simulink model "advanced_modelError"  (R2023a)
settings: Solver=ode1  StartTime=0  StopTime=1200  FixedStep=0.002  RelTol=1e-3  EnableMultiTasking=on
values from neighbouring files (symbols this model uses):
  angleLim = pi/3    (= 1.0471975512)    [modelCompPlot.m]
  B = b*L*(K_v)^2 /J_xx    (= 0.042375883612)    [advanced_model_setup.m]    (also in brusselator.m = 2.15; cycle_detection.m = img2; cycle_detection_start.m = img2; demonstrateDetections.m = 2.15)
  cycleGain = 0.1    [advanced_model_setup.m]
  f_p = 1.3    [advanced_model_setup.m]    (also in modelCompPlot.m)
  f_r = 0.4    [advanced_model_setup.m]    (also in modelCompPlot.m)
  f_y = 0.175    [advanced_model_setup.m]    (also in modelCompPlot.m)
  g_p = 10.5    [advanced_model_setup.m]    (also in modelCompPlot.m)
  g_r = 5.2    [advanced_model_setup.m]    (also in modelCompPlot.m)
  I_xx = 0.0522    [advanced_model_setup.m]    (also in modelCompPlot.m; set_model_params.m; solveSyms3d_2.m = evalin('base', 'I_xx'))
  I_yy = 0.0522    [advanced_model_setup.m]    (also in modelCompPlot.m; set_model_params.m; solveSyms3d_2.m = evalin('base', 'I_yy'))
  I_zz = 0.1104    [advanced_model_setup.m]    (also in modelCompPlot.m; set_model_params.m; solveSyms3d_2.m = evalin('base', 'I_zz'))
  J = (J_yy - J_zz)/J_xx    (= -1)    [advanced_model_setup.m]    (also in modelCompPlot.m)
  J_r = J_inertia/J_xx    (= 0.00108695652174)    [advanced_model_setup.m]    (also in modelCompPlot.m; solveSyms3d.m = evalin('base', 'J_r'))
  Jp = 2*Jeq_prop    (= 0.0552224595625)    [modelCompPlot.m]    (also in set_model_params.m)
  Jr = 2*Jeq_prop    (= 0.0552224595625)    [modelCompPlot.m]    (also in set_model_params.m)
  k_T = 0.1188    [advanced_model_setup.m]    (also in modelCompPlot.m; set_model_params.m; solveSyms3d_2.m = evalin('base', 'k_T'))
  K_v = 54.945    [advanced_model_setup.m]    (also in modelCompPlot.m; solveSyms3d.m = evalin('base', 'K_v'))
  kd = 0.5    [advanced_model_setup.m]
  Kf = 0.1188    [modelCompPlot.m]    (also in set_model_params.m)
  kfr_p = 0.4*u2line/x5line    (= 0.285774113641)    [advanced_model_setup.m]    (also in modelCompPlot.m; set_model_params.m)
  kfr_r = 0.4*u1line/x4line    (= 0.285774113641)    [advanced_model_setup.m]    (also in modelCompPlot.m; set_model_params.m)
  L = 0.1969    [advanced_model_setup.m]    (also in modelCompPlot.m; set_model_params.m = 0.19685)
  l_a = 0.1968    [advanced_model_setup.m]    (also in modelCompPlot.m; set_model_params.m; solveSyms3d_2.m = evalin('base', 'l_a'))
  r = 0.2    [advanced_model_setup.m]    (also in gainScheduling.m = evalin('base', 'r'))
  sigma = 0    [modelCompPlot.m]
  skew = 1    [advanced_model_setup.m]
  V_bias = 12    [advanced_model_setup.m]    (also in modelCompPlot.m; set_model_params.m; solveSyms3d.m = evalin('base', 'V_bias'))
  velMax = 1000    [advanced_model_setup.m]
  VMAX_AMP = 24    [advanced_model_setup.m]    (also in modelCompPlot.m; set_model_params.m)
  wcf = 2 * pi * 20    (= 125.663706144)    [advanced_model_setup.m]    (also in modelCompPlot.m; set_model_params.m)
  Y = d*(K_v)^2 /J_zz    (= 0.0032609614876)    [advanced_model_setup.m]    (also in modelCompPlot.m; solveSyms3d.m = evalin('base', 'Y'))
  zetaf = 0.6    [advanced_model_setup.m]    (also in modelCompPlot.m; set_model_params.m)
libraries: simulink_extras x4, dspsrcs4 x1
settings Model: ExtModeTrigDuration=10000  Creator=kille  LastModifiedBy=Jacob
settings SolverCC: PositivePriorityOrder=on  AutoInsertRateTranBlk=on
settings DataIOCC: ReturnWorkspaceOutputs=off
settings OptimizationCC: LifeSpan=inf
settings DebuggingCC: UnconnectedInputMsg=warning  UnconnectedOutputMsg=warning  UnconnectedLineMsg=warning  ArithmeticOperatorsInVariantConditions=warning
settings ModelReferenceCC: EnableRefExpFcnMdlSchedulingChecks=on
settings SFSimCC: SimUseLocalCustomCode=off  CustomCodeUndefinedFunction=UseInterfaceOnly
settings RTWCC: Description=QUARC Win64 Target  SystemTargetFile=quarc_win64.tlc  TemplateMakefile=quarc_default_tmf  RTWUseLocalCustomCode=off
settings CodeAppCC: StateflowObjectComments=on
settings STFCustomTargetCC: TargetPreCompLibLocation=C:\PROGRA~3\QUARC\lib\2016a\win64\release  UseToolchainInfoCompliant=off  SystemTargetFile=quarc_win64.tlc
settings GRTTargetCC: TargetPreCompLibLocation=C:\PROGRA~3\QUARC\lib\2016a\win64\release  ParMdlRefBuildCompliant=off  CompOptLevelCompliant=off  CombineOutputUpdateFcns=off  MatFileLogging=off  CPPClassGenCompliant=off  GRTInterface=on  UseToolchainInfoCompliant=off  ExtMode=on  ExtModeMexFile=quarc_comm
settings ConfigComp: CovMetricSettings=dswe

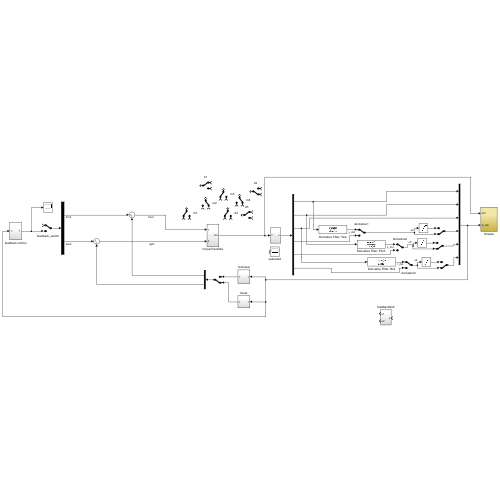
[thumbnail: Simulink's stored preview of the top-level diagram]
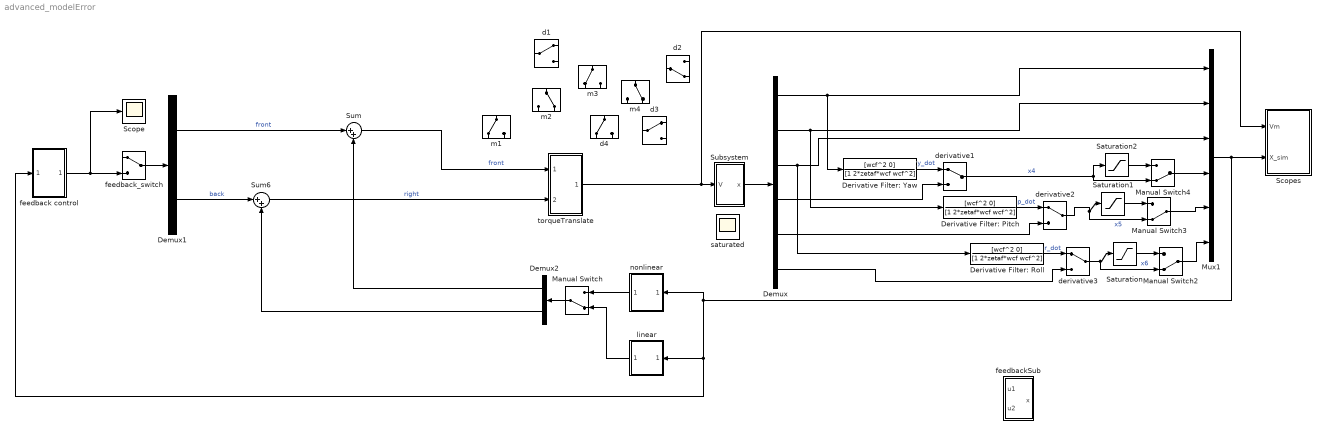
== system advanced_modelError ==
  Demux : Demux  Outputs=6
  Demux1 : Demux  Outputs=2
  Demux2 : Demux  Outputs=2
  Derivative Filter: Pitch : TransferFcn  Numerator=[wcf^2 0]  Denominator=[1 2*zetaf*wcf wcf^2]
  Derivative Filter: Roll : TransferFcn  Numerator=[wcf^2 0]  Denominator=[1 2*zetaf*wcf wcf^2]
  Derivative Filter: Yaw : TransferFcn  Numerator=[wcf^2 0]  Denominator=[1 2*zetaf*wcf wcf^2]
  Manual Switch{,2..4} (4 alike) : ManualSwitch  CurrentSetting=0
  Mux1 : Mux  Inputs=6
  Saturation : Saturate  UpperLimit=velMax  LowerLimit=-velMax
  Saturation1 : Saturate  UpperLimit=velMax  LowerLimit=-velMax
  Saturation2 : Saturate  UpperLimit=velMax  LowerLimit=-velMax
  Scope : Scope
  Scopes : Subsystem
  Subsystem : Subsystem
  Sum : Sum  Inputs=|++
  Sum6 : Sum  Inputs=|++
  d1 : ManualSwitch
  d2 : ManualSwitch  CurrentSetting=0
  d3 : ManualSwitch
  d4 : ManualSwitch
  derivative1 : ManualSwitch
  derivative2 : ManualSwitch
  derivative3 : ManualSwitch
  feedback control : Subsystem
  feedbackSub : Subsystem
  feedback_switch : ManualSwitch
  linear : Subsystem
  m1 : ManualSwitch
  m2 : ManualSwitch  CurrentSetting=0
  m3 : ManualSwitch
  m4 : ManualSwitch  CurrentSetting=0
  nonlinear : Subsystem
  saturated : Scope
  torqueTranslate : Subsystem
  wires:
  Sum6/1 -> torqueTranslate/2(Input)  "right"
  Sum/1 -> torqueTranslate/1(In1)  "front"
  derivative2/1 -> Manual Switch3/2, Saturation1/1  "x5"
  Derivative Filter: Pitch/1 -> derivative2/1  "p_dot"
  Saturation2/1 -> Manual Switch4/1
  Saturation1/1 -> Manual Switch3/1
  Saturation/1 -> Manual Switch2/1
  Demux/4 -> derivative1/2
  derivative1/1 -> Saturation2/1, Manual Switch4/2  "x4"
  derivative3/1 -> Manual Switch2/2, Saturation/1  "x6"
  Derivative Filter: Roll/1 -> derivative3/1  "r_dot"
  Derivative Filter: Yaw/1 -> derivative1/1  "y_dot"
  Subsystem/1(x) -> Demux/1
  Manual Switch4/1 -> Mux1/4
  Manual Switch3/1 -> Mux1/5
  Manual Switch2/1 -> Mux1/6
  Demux/1 -> Derivative Filter: Yaw/1, Mux1/1
  Demux/2 -> Derivative Filter: Pitch/1, Mux1/2
  Demux/3 -> Derivative Filter: Roll/1, Mux1/3
  Demux/5 -> derivative2/2
  Demux/6 -> derivative3/2
  Demux1/1 -> Sum/1  "front"
  Demux1/2 -> Sum6/1  "back"
  feedback_switch/1 -> Demux1/1
  feedback control/1(Out1) -> Scope/1, feedback_switch/2
  Demux2/1 -> Sum/2
  Demux2/2 -> Sum6/2
  Manual Switch/1 -> Demux2/1
  nonlinear/1(Out1) -> Manual Switch/1
  linear/1(Out1) -> Manual Switch/2
  Mux1/1 -> Scopes/2(X_sim), linear/1(Input), feedback control/1(In1), nonlinear/1(Input)
  torqueTranslate/1(Vm) -> Scopes/1(Vm), Subsystem/1(V)

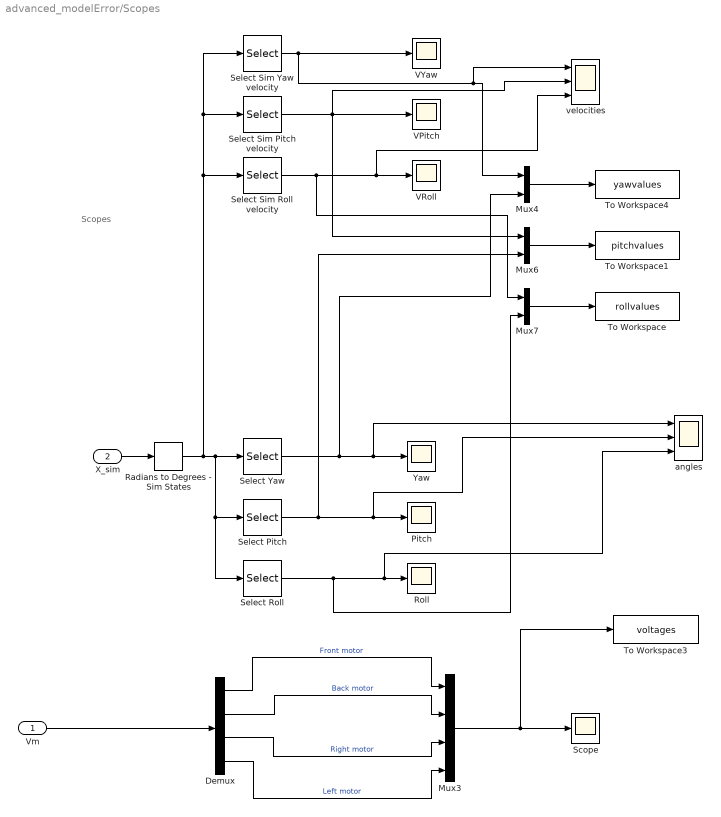
== system advanced_modelError/Scopes ==
  note: Scopes
  Vm : Inport
  X_sim : Inport  Port=2
  Demux : Demux
  Mux3 : Mux
  Mux4 : Mux  Inputs=2
  Mux6 : Mux  Inputs=2
  Mux7 : Mux  Inputs=2
  Pitch : Scope
  Radians to Degrees - Sim States : simulink_extras/Transformations/Radians to Degrees
  Roll : Scope
  Scope : Scope
  Select Pitch : Selector  InputPortWidth=6  IndexOptions=Index vector (dialog)  Indices=2  OutputSizes=1
  Select Roll : Selector  InputPortWidth=6  IndexOptions=Index vector (dialog)  Indices=3  OutputSizes=1
  Select Sim Pitch velocity : Selector  InputPortWidth=6  IndexOptions=Index vector (dialog)  Indices=5  OutputSizes=1
  Select Sim Roll velocity : Selector  InputPortWidth=6  IndexOptions=Index vector (dialog)  Indices=6  OutputSizes=1
  Select Sim Yaw velocity : Selector  InputPortWidth=6  IndexOptions=Index vector (dialog)  Indices=4  OutputSizes=1
  Select Yaw : Selector  InputPortWidth=6  IndexOptions=Index vector (dialog)  Indices=1  OutputSizes=1
  To Workspace : ToWorkspace  VariableName=rollvalues  SampleTime=-1
  To Workspace1 : ToWorkspace  VariableName=pitchvalues  SampleTime=-1
  To Workspace3 : ToWorkspace  VariableName=voltages  SampleTime=-1
  To Workspace4 : ToWorkspace  VariableName=yawvalues  SampleTime=-1
  VPitch : Scope
  VRoll : Scope
  VYaw : Scope
  Yaw : Scope
  angles : Scope  NumInputPorts=3
  velocities : Scope  NumInputPorts=3
  wires:
  Select Roll/1 -> angles/3, Roll/1, Mux7/2
  Radians to Degrees - Sim States/1 -> Select Sim Roll velocity/1, Select Sim Pitch velocity/1, Select Sim Yaw velocity/1, Select Roll/1, Select Pitch/1, Select Yaw/1
  Select Pitch/1 -> angles/2, Pitch/1, Mux6/2
  X_sim/1 -> Radians to Degrees - Sim States/1
  Demux/1 -> Mux3/1  "Front motor"
  Demux/2 -> Mux3/2  "Back motor"
  Demux/3 -> Mux3/3  "Right motor"
  Demux/4 -> Mux3/4  "Left motor"
  Vm/1 -> Demux/1
  Select Sim Yaw velocity/1 -> VYaw/1, velocities/1, Mux4/1
  Select Sim Roll velocity/1 -> velocities/3, VRoll/1, Mux7/1
  Select Sim Pitch velocity/1 -> Mux6/1, velocities/2, VPitch/1
  Mux4/1 -> To Workspace4/1
  Mux6/1 -> To Workspace1/1
  Mux7/1 -> To Workspace/1
  Mux3/1 -> To Workspace3/1, Scope/1
  Select Yaw/1 -> angles/1, Yaw/1, Mux4/2

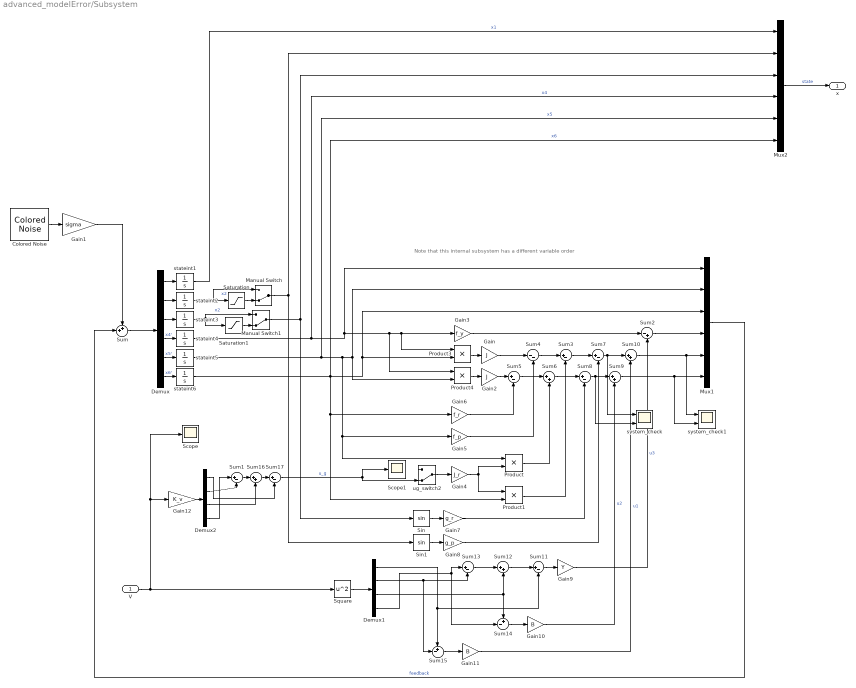
== system advanced_modelError/Subsystem ==
  note: Note that this internal subsystem has a different variable order
  V : Inport
  Colored Noise : dspsrcs4/Colored Noise  Color=white  InverseFrequencyPower=1  BoundedOutput=off  NumChannels=6  OutputDataType=double  SamplesPerFrame=1  SampleTime=1  RandomStream=mt19937ar with seed  Seed=67  SimulateUsing=Interpreted execution
  Demux : Demux  Outputs=6
  Demux1 : Demux
  Demux2 : Demux
  Gain : Gain  Gain=J
  Gain1 : Gain  Gain=sigma
  Gain10 : Gain  Gain=B
  Gain11 : Gain  Gain=B
  Gain12 : Gain  Gain=K_v
  Gain2 : Gain  Gain=J
  Gain3 : Gain  Gain=f_y
  Gain4 : Gain  Gain=J_r
  Gain5 : Gain  Gain=f_p
  Gain6 : Gain  Gain=f_r
  Gain7 : Gain  Gain=g_r
  Gain8 : Gain  Gain=g_p
  Gain9 : Gain  Gain=Y
  Manual Switch : ManualSwitch  CurrentSetting=0
  Manual Switch1 : ManualSwitch  CurrentSetting=0
  Mux1 : Mux  Inputs=6
  Mux2 : Mux  Inputs=6
  Product{,1,3..4} (4 alike) : Product
  Saturation : Saturate  UpperLimit=angleLim  LowerLimit=-angleLim
  Saturation1 : Saturate  UpperLimit=angleLim  LowerLimit=-angleLim
  Scope : Scope
  Scope1 : Scope
  Sin : Trigonometry
  Sin1 : Trigonometry
  Square : Math  Operator=square
  Sum : Sum  Inputs=++|
  Sum{1,3,5,7..8,11,13,17} (8 alike) : Sum  Inputs=|+-
  Sum{6,9..10,12,16} (5 alike) : Sum  Inputs=|++
  Sum14 : Sum  Inputs=+-|
  Sum15 : Sum  Inputs=+-|
  Sum2 : Sum  Inputs=|-+
  Sum4 : Sum  Inputs=|--
  stateint1 : Integrator  InitialCondition=0.034907
  stateint2 : Integrator  InitialCondition=0.034907
  stateint3 : Integrator  InitialCondition=0.034907
  stateint4 : Integrator
  stateint5 : Integrator
  stateint6 : Integrator
  system_check : Scope  NumInputPorts=2
  system_check1 : Scope  NumInputPorts=2
  ug_switch2 : ManualSwitch  CurrentSetting=0
  x : Outport
  wires:
  stateint5/1 -> Mux2/5, Gain5/1, Product/1, Mux1/2, Product4/2  "x5"
  stateint4/1 -> Mux2/4, Mux1/1, Product4/1, Product3/1, Gain3/1  "x4"
  Demux/1 -> stateint1/1
  stateint6/1 -> Mux2/6, Gain6/1, Product1/2, Mux1/3, Product3/2  "x6"
  Demux/6 -> stateint6/1  "x6'"
  Demux/5 -> stateint5/1  "x5'"
  Demux/2 -> stateint2/1
  Demux/3 -> stateint3/1
  Demux/4 -> stateint4/1  "x4'"
  Product3/1 -> Gain/1
  Product4/1 -> Gain2/1
  Colored Noise/1 -> Gain1/1
  Sum/1 -> Demux/1
  Gain1/1 -> Sum/1
  Gain3/1 -> Sum2/1
  Gain4/1 -> Product1/1, Product/2
  Sum17/1 -> ug_switch2/2, Scope1/1  "u_g"
  Gain/1 -> Sum4/1
  Gain2/1 -> Sum5/1
  Gain6/1 -> Sum5/2
  Gain5/1 -> Sum4/2
  Sum5/1 -> Sum6/1
  Product/1 -> Sum6/2
  Sum4/1 -> Sum3/1
  Sum6/1 -> Sum8/1
  Sum3/1 -> Sum7/1
  Gain7/1 -> Sum8/2
  Gain8/1 -> Sum7/2
  Sin/1 -> Gain7/1
  Sin1/1 -> Gain8/1
  Sum8/1 -> system_check/2, Sum9/1
  Sum7/1 -> system_check/1, Sum10/1
  Sum11/1 -> Gain9/1
  Gain9/1 -> Sum2/2  "u3"
  Square/1 -> Demux1/1
  Sum12/1 -> Sum11/1
  Sum13/1 -> Sum12/1
  Demux1/4 -> Sum13/1, Sum14/2
  Demux1/2 -> Sum13/2, Sum15/2
  Demux1/3 -> Sum12/2, Sum14/1
  Demux1/1 -> Sum15/1, Sum11/2
  Sum14/1 -> Gain10/1
  Sum15/1 -> Gain11/1
  Gain10/1 -> Sum9/2  "u2"
  Gain11/1 -> Sum10/2  "u1"
  Mux1/1 -> Sum/2  "feedback"
  V/1 -> Square/1, Scope/1, Gain12/1
  Gain12/1 -> Demux2/1
  Sum1/1 -> Sum16/1
  Sum16/1 -> Sum17/1
  Demux2/2 -> Sum1/2
  Demux2/3 -> Sum16/2
  Sum10/1 -> system_check1/1, Mux1/5
  Sum2/1 -> Mux1/4
  stateint2/1 -> Manual Switch/1, Saturation/1  "x2"
  Product1/1 -> Sum3/2
  Demux2/4 -> Sum1/1
  Demux2/1 -> Sum17/2
  stateint1/1 -> Mux2/1  "x1"
  Mux2/1 -> x/1  "state"
  Sum9/1 -> system_check1/2, Mux1/6
  ug_switch2/1 -> Gain4/1
  Manual Switch/1 -> Sin1/1, Mux2/2
  Saturation/1 -> Manual Switch/2
  Manual Switch1/1 -> Mux2/3, Sin/1
  stateint3/1 -> Saturation1/1, Manual Switch1/1  "x2"
  Saturation1/1 -> Manual Switch1/2

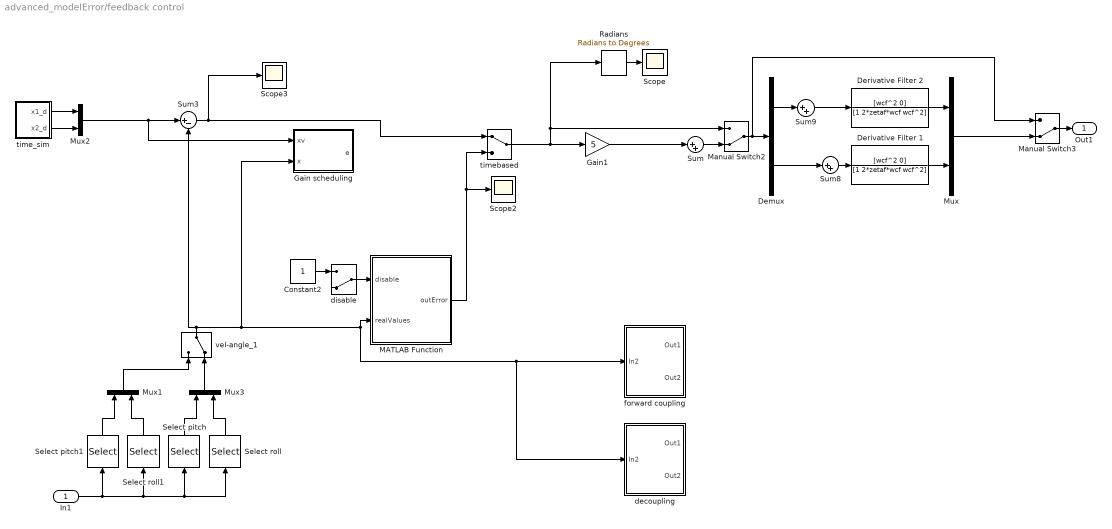
== system advanced_modelError/feedback control ==
  In1 : Inport
  Constant2 : Constant
  Demux : Demux  Outputs=2
  Derivative Filter 1 : TransferFcn  Numerator=[wcf^2 0]  Denominator=[1 2*zetaf*wcf wcf^2]
  Derivative Filter 2 : TransferFcn  Numerator=[wcf^2 0]  Denominator=[1 2*zetaf*wcf wcf^2]
  Gain scheduling : MATLAB Function  TreatAsAtomicUnit=on
  Gain1 : Gain  Gain=5
  MATLAB Function : MATLAB Function  TreatAsAtomicUnit=on
  Manual Switch2 : ManualSwitch  CurrentSetting=0
  Manual Switch3 : ManualSwitch  CurrentSetting=0
  Mux{,1..3} (4 alike) : Mux  Inputs=2
  Radians : simulink_extras/Transformations/Radians to Degrees
  Scope : Scope
  Scope2 : Scope
  Scope3 : Scope
  Select pitch : Selector  InputPortWidth=6  IndexOptions=Index vector (dialog)  Indices=2  OutputSizes=1
  Select pitch1 : Selector  InputPortWidth=6  IndexOptions=Index vector (dialog)  Indices=5  OutputSizes=1
  Select roll : Selector  InputPortWidth=6  IndexOptions=Index vector (dialog)  Indices=3  OutputSizes=1
  Select roll1 : Selector  InputPortWidth=6  IndexOptions=Index vector (dialog)  Indices=6  OutputSizes=1
  Sum : Sum  Inputs=|++
  Sum3 : Sum  Inputs=|+-
  Sum8 : Sum  Inputs=|++
  Sum9 : Sum  Inputs=|++
  decoupling : Subsystem
  disable : ManualSwitch  CurrentSetting=0
  forward coupling : Subsystem
  time_sim : Subsystem
  timebased : ManualSwitch
  vel-angle_1 : ManualSwitch  CurrentSetting=0
  Out1 : Outport
  wires:
  In1/1 -> Select roll/1, Select pitch/1, Select roll1/1, Select pitch1/1
  Select pitch/1 -> Mux3/1
  time_sim/1(x1_d) -> Mux2/1
  time_sim/2(x2_d) -> Mux2/2
  Select roll/1 -> Mux3/2
  MATLAB Function/1(outError) -> Scope2/1, timebased/2
  Sum/1 -> Manual Switch2/2
  Radians/1 -> Scope/1
  disable/1 -> MATLAB Function/1(disable)
  Constant2/1 -> disable/1
  Select roll1/1 -> Mux1/2
  Select pitch1/1 -> Mux1/1
  Mux1/1 -> vel-angle_1/1
  Mux3/1 -> vel-angle_1/2
  Mux2/1 -> Gain scheduling/1(xv), Sum3/1
  Derivative Filter 2/1 -> Mux/1
  Derivative Filter 1/1 -> Mux/2
  Manual Switch2/1 -> Manual Switch3/1, Demux/1
  Manual Switch3/1 -> Out1/1
  Demux/2 -> Sum8/1
  Mux/1 -> Manual Switch3/2
  vel-angle_1/1 -> Sum3/2, Gain scheduling/2(x), MATLAB Function/2(realValues), decoupling/1(In2), forward coupling/1(In2)
  Sum8/1 -> Derivative Filter 1/1
  Sum9/1 -> Derivative Filter 2/1
  Demux/1 -> Sum9/1
  Sum3/1 -> Scope3/1, timebased/1
  Gain1/1 -> Sum/1
  timebased/1 -> Manual Switch2/1, Radians/1, Gain1/1

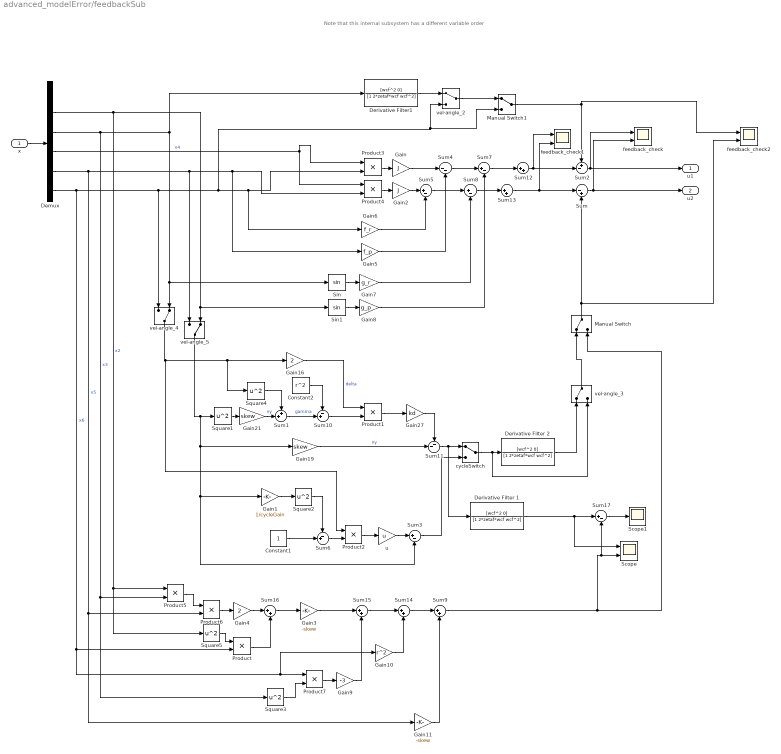
== system advanced_modelError/feedbackSub ==
  note: Note that this internal subsystem has a different variable order
  x : Inport
  Constant1 : Constant
  Constant2 : Constant  Value=r^2
  Demux : Demux  Outputs=6
  Derivative Filter 1 : TransferFcn  Numerator=[wcf^2 0]  Denominator=[1 2*zetaf*wcf wcf^2]
  Derivative Filter 2 : TransferFcn  Numerator=[wcf^2 0]  Denominator=[1 2*zetaf*wcf wcf^2]
  Derivative Filter1 : TransferFcn  Numerator=[wcf^2 0]  Denominator=[1 2*zetaf*wcf wcf^2]
  Gain : Gain  Gain=J
  Gain1 : Gain  Gain=1/cycleGain
  Gain10 : Gain  Gain=r^2
  Gain11 : Gain  Gain=-skew
  Gain16 : Gain  Gain=2
  Gain19 : Gain  Gain=skew
  Gain2 : Gain  Gain=J
  Gain21 : Gain  Gain=skew
  Gain27 : Gain  Gain=kd
  Gain3 : Gain  Gain=-skew
  Gain4 : Gain  Gain=2
  Gain5 : Gain  Gain=f_p
  Gain6 : Gain  Gain=f_r
  Gain7 : Gain  Gain=g_r
  Gain8 : Gain  Gain=g_p
  Gain9 : Gain  Gain=-3
  Manual Switch : ManualSwitch
  Manual Switch1 : ManualSwitch
  Product{,1..7} (8 alike) : Product
  Scope : Scope  NumInputPorts=2
  Scope1 : Scope
  Sin : Trigonometry
  Sin1 : Trigonometry
  Square{1..5} (5 alike) : Math  Operator=square
  Sum : Sum  Inputs=|-+
  Sum1 : Sum  Inputs=++|
  Sum10 : Sum  Inputs=-+|
  Sum11 : Sum  Inputs=--|
  Sum{9,12..16} (6 alike) : Sum  Inputs=|++
  Sum{3,5,7..8,17} (5 alike) : Sum  Inputs=|+-
  Sum2 : Sum  Inputs=+-|
  Sum4 : Sum  Inputs=|--
  Sum6 : Sum  Inputs=-+|
  cycleSwitch : ManualSwitch
  feedback_check : Scope  NumInputPorts=2
  feedback_check1 : Scope  NumInputPorts=2
  feedback_check2 : Scope  NumInputPorts=2
  u : Gain  Gain=u
  vel-angle_2 : ManualSwitch
  vel-angle_3 : ManualSwitch
  vel-angle_4 : ManualSwitch  CurrentSetting=0
  vel-angle_5 : ManualSwitch  CurrentSetting=0
  u1 : Outport
  u2 : Outport  Port=2
  wires:
  Demux/4 -> Product3/1, Product4/1  "x4"
  Product3/1 -> Gain/1
  Product4/1 -> Gain2/1
  Gain/1 -> Sum4/1
  Gain2/1 -> Sum5/1
  Gain6/1 -> Sum5/2
  Gain5/1 -> Sum4/2
  Sum4/1 -> Sum7/1
  Gain7/1 -> Sum8/2
  Gain8/1 -> Sum7/2
  Sin/1 -> Gain7/1
  Sin1/1 -> Gain8/1
  Demux/3 -> Square3/1, Product5/2, Derivative Filter1/1, Sin/1, vel-angle_4/2  "x3"
  Sum5/1 -> Sum8/1
  Derivative Filter 2/1 -> vel-angle_3/1
  Square1/1 -> Gain21/1
  Product1/1 -> Gain27/1
  Sum1/1 -> Sum10/2  "gamma"
  Constant2/1 -> Sum10/1
  Sum10/1 -> Product1/2
  Gain16/1 -> Product1/1  "delta"
  Gain21/1 -> Sum1/2  "ny"
  Square4/1 -> Sum1/1
  Gain27/1 -> Sum11/1
  Gain19/1 -> Sum11/2  "ny"
  Derivative Filter1/1 -> vel-angle_2/1
  Sum2/1 -> u1/1, feedback_check/1
  Sum/1 -> u2/1, feedback_check/2
  Sum6/1 -> Product2/2
  Demux/2 -> Sin1/1, vel-angle_5/2, Product5/1, Square5/1  "x2"
  Gain1/1 -> Square2/1
  u/1 -> Sum3/1
  Product2/1 -> u/1
  Square2/1 -> Sum6/1
  Constant1/1 -> Sum6/2
  Sum11/1 -> Derivative Filter 1/1, cycleSwitch/1
  cycleSwitch/1 -> vel-angle_3/2, Derivative Filter 2/1
  Sum3/1 -> cycleSwitch/2
  Demux/5 -> Gain11/1, Product6/2, Product4/2, Gain5/1, vel-angle_5/1  "x5"
  Demux/6 -> Gain10/1, Product7/1, Product/2, vel-angle_4/1, Manual Switch1/2, vel-angle_2/2, Gain6/1, Product3/2  "x6"
  Sum7/1 -> Sum12/1
  Sum8/1 -> Sum13/1
  Sum12/1 -> feedback_check1/1, Sum2/2
  Sum13/1 -> feedback_check1/2, Sum/1
  x/1 -> Demux/1
  vel-angle_4/1 -> Product2/1, Square4/1, Gain16/1
  vel-angle_5/1 -> Gain19/1, Gain1/1, Sum3/2, Square1/1
  Sum15/1 -> Sum14/1
  Sum14/1 -> Sum9/1
  Gain3/1 -> Sum15/1
  Sum16/1 -> Gain3/1
  Gain4/1 -> Sum16/1
  Product/1 -> Sum16/2
  Product6/1 -> Gain4/1
  Product5/1 -> Product6/1
  Product7/1 -> Gain9/1
  Gain9/1 -> Sum15/2
  Square3/1 -> Product7/2
  Gain10/1 -> Sum14/2
  Gain11/1 -> Sum9/2
  Square5/1 -> Product/1
  Sum17/1 -> Scope1/1
  Sum9/1 -> Scope/2, Sum17/2, Manual Switch/2
  Derivative Filter 1/1 -> Scope/1, Sum17/1
  Manual Switch/1 -> Sum/2, feedback_check2/2
  vel-angle_3/1 -> Manual Switch/1
  Manual Switch1/1 -> feedback_check2/1, Sum2/1
  vel-angle_2/1 -> Manual Switch1/1

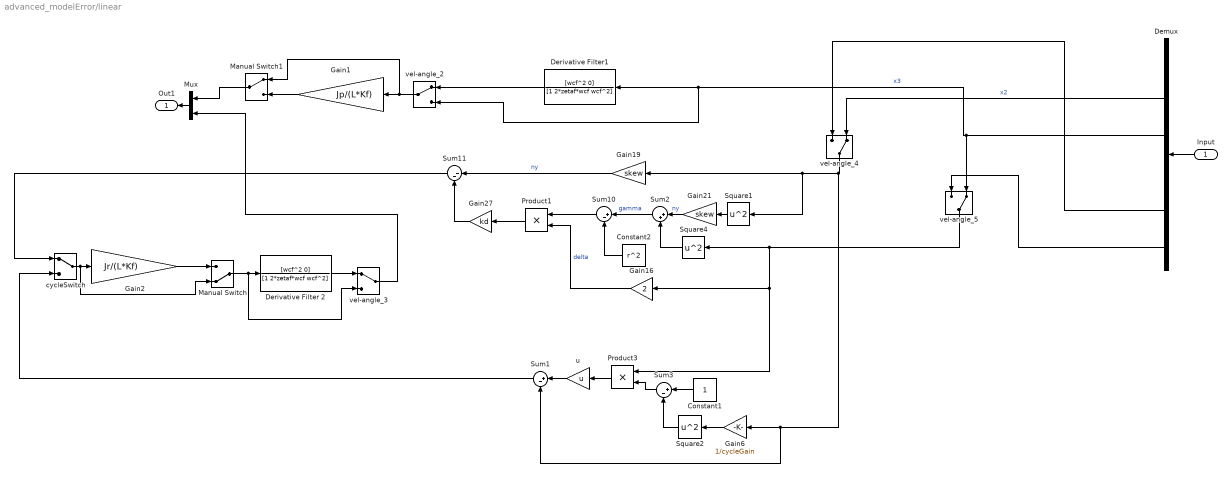
== system advanced_modelError/linear ==
  Input : Inport
  Constant1 : Constant
  Constant2 : Constant  Value=r^2
  Demux : Demux  Outputs=6
  Derivative Filter 2 : TransferFcn  Numerator=[wcf^2 0]  Denominator=[1 2*zetaf*wcf wcf^2]
  Derivative Filter1 : TransferFcn  Numerator=[wcf^2 0]  Denominator=[1 2*zetaf*wcf wcf^2]
  Gain1 : Gain  Gain=Jp/(L*Kf)
  Gain16 : Gain  Gain=2
  Gain19 : Gain  Gain=skew
  Gain2 : Gain  Gain=Jr/(L*Kf)
  Gain21 : Gain  Gain=skew
  Gain27 : Gain  Gain=kd
  Gain6 : Gain  Gain=1/cycleGain
  Manual Switch : ManualSwitch  CurrentSetting=0
  Manual Switch1 : ManualSwitch
  Mux : Mux  Inputs=2
  Product1 : Product
  Product3 : Product
  Square1 : Math  Operator=square
  Square2 : Math  Operator=square
  Square4 : Math  Operator=square
  Sum1 : Sum  Inputs=|+-
  Sum10 : Sum  Inputs=|+-
  Sum11 : Sum  Inputs=|--
  Sum2 : Sum  Inputs=|++
  Sum3 : Sum  Inputs=|+-
  cycleSwitch : ManualSwitch
  u : Gain  Gain=u
  vel-angle_2 : ManualSwitch
  vel-angle_3 : ManualSwitch
  vel-angle_4 : ManualSwitch  CurrentSetting=0
  vel-angle_5 : ManualSwitch  CurrentSetting=0
  Out1 : Outport
  wires:
  Square1/1 -> Gain21/1
  Product1/1 -> Gain27/1
  Square4/1 -> Sum2/2
  Gain19/1 -> Sum11/1  "ny"
  Sum2/1 -> Sum10/1  "gamma"
  Gain16/1 -> Product1/2  "delta"
  Sum10/1 -> Product1/1
  Gain27/1 -> Sum11/2
  Gain21/1 -> Sum2/1  "ny"
  Constant2/1 -> Sum10/2
  Sum1/1 -> cycleSwitch/2
  Demux/3 -> vel-angle_2/2, Derivative Filter1/1, vel-angle_5/2  "x3"
  u/1 -> Sum1/1
  Gain6/1 -> Square2/1
  Product3/1 -> u/1
  Constant1/1 -> Sum3/1
  Sum3/1 -> Product3/2
  Square2/1 -> Sum3/2
  Demux/2 -> vel-angle_4/2  "x2"
  Sum11/1 -> cycleSwitch/1
  Derivative Filter1/1 -> vel-angle_2/1
  vel-angle_2/1 -> Manual Switch1/1, Gain1/1
  cycleSwitch/1 -> Manual Switch/2, Gain2/1
  Derivative Filter 2/1 -> vel-angle_3/1
  Input/1 -> Demux/1
  vel-angle_4/1 -> Gain6/1, Sum1/2, Square1/1, Gain19/1
  Demux/5 -> vel-angle_4/1
  vel-angle_5/1 -> Product3/1, Gain16/1, Square4/1
  Demux/6 -> vel-angle_5/1
  Gain2/1 -> Manual Switch/1
  Manual Switch/1 -> vel-angle_3/2, Derivative Filter 2/1
  Gain1/1 -> Manual Switch1/2
  Manual Switch1/1 -> Mux/1
  vel-angle_3/1 -> Mux/2
  Mux/1 -> Out1/1

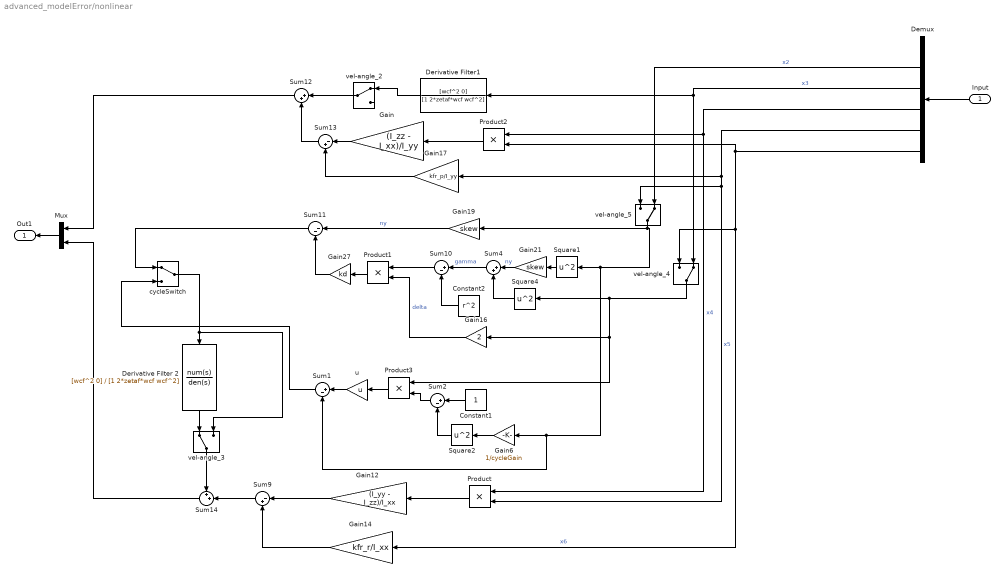
== system advanced_modelError/nonlinear ==
  Input : Inport
  Constant1 : Constant
  Constant2 : Constant  Value=r^2
  Demux : Demux  Outputs=6
  Derivative Filter 2 : TransferFcn  Numerator=[wcf^2 0]  Denominator=[1 2*zetaf*wcf wcf^2]
  Derivative Filter1 : TransferFcn  Numerator=[wcf^2 0]  Denominator=[1 2*zetaf*wcf wcf^2]
  Gain : Gain  Gain=(I_zz - I_xx)/I_yy
  Gain12 : Gain  Gain=(I_yy - I_zz)/I_xx
  Gain14 : Gain  Gain=kfr_r/I_xx
  Gain16 : Gain  Gain=2
  Gain17 : Gain  Gain=kfr_p/I_yy
  Gain19 : Gain  Gain=skew
  Gain21 : Gain  Gain=skew
  Gain27 : Gain  Gain=kd
  Gain6 : Gain  Gain=1/cycleGain
  Mux : Mux  Inputs=2
  Product{,1..3} (4 alike) : Product
  Square1 : Math  Operator=square
  Square2 : Math  Operator=square
  Square4 : Math  Operator=square
  Sum1 : Sum  Inputs=|+-
  Sum10 : Sum  Inputs=|+-
  Sum11 : Sum  Inputs=|--
  Sum12 : Sum  Inputs=|++
  Sum13 : Sum  Inputs=|-+
  Sum14 : Sum  Inputs=++|
  Sum2 : Sum  Inputs=|+-
  Sum4 : Sum  Inputs=|++
  Sum9 : Sum  Inputs=|-+
  cycleSwitch : ManualSwitch
  u : Gain  Gain=u
  vel-angle_2 : ManualSwitch
  vel-angle_3 : ManualSwitch
  vel-angle_4 : ManualSwitch  CurrentSetting=0
  vel-angle_5 : ManualSwitch  CurrentSetting=0
  Out1 : Outport
  wires:
  Derivative Filter1/1 -> vel-angle_2/1
  Gain17/1 -> Sum13/2
  Sum13/1 -> Sum12/2
  Demux/4 -> Product/1, Product2/1  "x4"
  Gain21/1 -> Sum4/1  "ny"
  Product2/1 -> Gain/1
  Demux/5 -> vel-angle_5/1, Product/2, Gain17/1  "x5"
  Gain27/1 -> Sum11/2
  Product/1 -> Gain12/1
  Constant2/1 -> Sum10/2
  Sum10/1 -> Product1/1
  Demux/6 -> vel-angle_4/1, Gain14/1, Product2/2  "x6"
  vel-angle_3/1 -> Sum14/1
  vel-angle_2/1 -> Sum12/1
  Sum4/1 -> Sum10/1  "gamma"
  Sum9/1 -> Sum14/2
  Square4/1 -> Sum4/2
  Gain12/1 -> Sum9/1
  Square1/1 -> Gain21/1
  Product1/1 -> Gain27/1
  Gain/1 -> Sum13/1
  Gain14/1 -> Sum9/2
  Sum12/1 -> Mux/1
  Gain19/1 -> Sum11/1  "ny"
  Gain16/1 -> Product1/2  "delta"
  Sum14/1 -> Mux/2
  Input/1 -> Demux/1
  Square2/1 -> Sum2/2
  Demux/2 -> vel-angle_5/2  "x2"
  Constant1/1 -> Sum2/1
  Sum2/1 -> Product3/2
  Product3/1 -> u/1
  Gain6/1 -> Square2/1
  Demux/3 -> Derivative Filter1/1, vel-angle_4/2  "x3"
  u/1 -> Sum1/1
  Sum11/1 -> cycleSwitch/1
  cycleSwitch/1 -> vel-angle_3/2, Derivative Filter 2/1
  Sum1/1 -> cycleSwitch/2
  vel-angle_4/1 -> Square4/1, Product3/1, Gain16/1
  vel-angle_5/1 -> Gain6/1, Sum1/2, Square1/1, Gain19/1
  Derivative Filter 2/1 -> vel-angle_3/1
  Mux/1 -> Out1/1

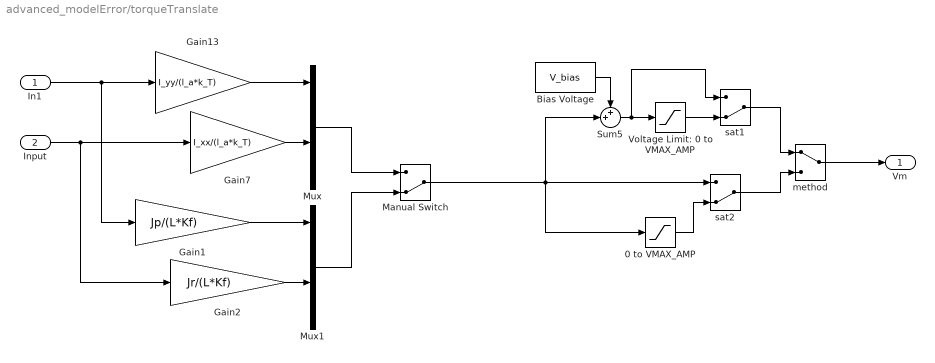
== system advanced_modelError/torqueTranslate ==
  In1 : Inport
  Input : Inport  Port=2
  0 to VMAX_AMP : Saturate  UpperLimit=VMAX_AMP  LowerLimit=0
  Bias Voltage : Constant  Value=V_bias
  Gain1 : Gain  Gain=Jp/(L*Kf)
  Gain13 : Gain  Gain=I_yy/(l_a*k_T)
  Gain2 : Gain  Gain=Jr/(L*Kf)
  Gain7 : Gain  Gain=I_xx/(l_a*k_T)
  Manual Switch : ManualSwitch  CurrentSetting=0
  Mux : Mux
  Mux1 : Mux
  Sum5 : Sum  Inputs=++|
  Voltage Limit: 0 to VMAX_AMP : Saturate  UpperLimit=VMAX_AMP  LowerLimit=0
  method : ManualSwitch  Tag=swt
  sat1 : ManualSwitch  CurrentSetting=0
  sat2 : ManualSwitch  CurrentSetting=0
  Vm : Outport
  wires:
  0 to VMAX_AMP/1 -> sat2/2
  Sum5/1 -> sat1/1, Voltage Limit: 0 to VMAX_AMP/1
  sat1/1 -> method/1
  Bias Voltage/1 -> Sum5/1
  Voltage Limit: 0 to VMAX_AMP/1 -> sat1/2
  sat2/1 -> method/2
  method/1 -> Vm/1
  Gain13/1 -> Mux/1
  In1/1 -> Gain13/1, Gain1/1
  Gain7/1 -> Mux/3
  Input/1 -> Gain7/1, Gain2/1
  Manual Switch/1 -> 0 to VMAX_AMP/1, Sum5/2, sat2/1
  Mux/1 -> Manual Switch/1
  Mux1/1 -> Manual Switch/2
  Gain1/1 -> Mux1/1
  Gain2/1 -> Mux1/3

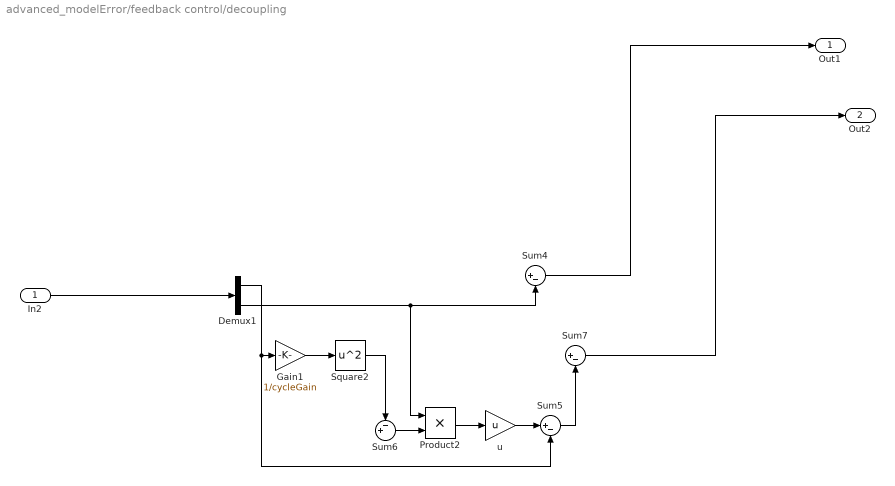
== system advanced_modelError/feedback control/decoupling ==
  In2 : Inport
  Demux1 : Demux  Outputs=2
  Gain1 : Gain  Gain=1/cycleGain
  Product2 : Product
  Square2 : Math  Operator=square
  Sum4 : Sum  Inputs=|+-
  Sum5 : Sum  Inputs=|+-
  Sum6 : Sum  Inputs=-+|
  Sum7 : Sum  Inputs=|+-
  u : Gain  Gain=u
  Out1 : Outport
  Out2 : Outport  Port=2
  wires:
  Sum5/1 -> Sum7/2
  Sum7/1 -> Out2/1
  Square2/1 -> Sum6/1
  u/1 -> Sum5/1
  Demux1/1 -> Sum5/2, Gain1/1
  Product2/1 -> u/1
  Demux1/2 -> Product2/1, Sum4/2
  Sum6/1 -> Product2/2
  Gain1/1 -> Square2/1
  In2/1 -> Demux1/1
  Sum4/1 -> Out1/1

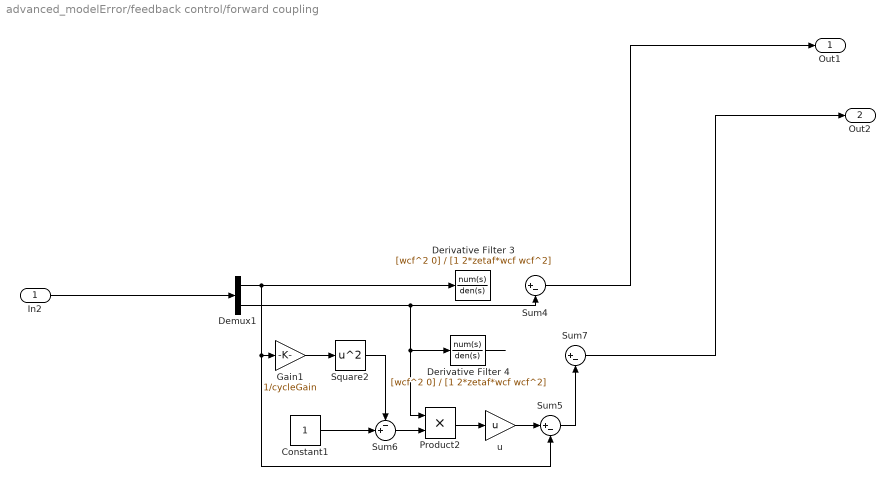
== system advanced_modelError/feedback control/forward coupling ==
  In2 : Inport
  Constant1 : Constant
  Demux1 : Demux  Outputs=2
  Derivative Filter 3 : TransferFcn  Numerator=[wcf^2 0]  Denominator=[1 2*zetaf*wcf wcf^2]
  Derivative Filter 4 : TransferFcn  Numerator=[wcf^2 0]  Denominator=[1 2*zetaf*wcf wcf^2]
  Gain1 : Gain  Gain=1/cycleGain
  Product2 : Product
  Square2 : Math  Operator=square
  Sum4 : Sum  Inputs=|+-
  Sum5 : Sum  Inputs=|+-
  Sum6 : Sum  Inputs=-+|
  Sum7 : Sum  Inputs=|+-
  u : Gain  Gain=u
  Out1 : Outport
  Out2 : Outport  Port=2
  wires:
  Sum5/1 -> Sum7/2
  Sum7/1 -> Out2/1
  Square2/1 -> Sum6/1
  u/1 -> Sum5/1
  Demux1/1 -> Sum5/2, Gain1/1, Derivative Filter 3/1
  Product2/1 -> u/1
  Demux1/2 -> Product2/1, Derivative Filter 4/1, Sum4/2
  Sum6/1 -> Product2/2
  ? -> Sum7/1
  Constant1/1 -> Sum6/2
  Gain1/1 -> Square2/1
  In2/1 -> Demux1/1
  Sum4/1 -> Out1/1
  Derivative Filter 4/1 -> ?

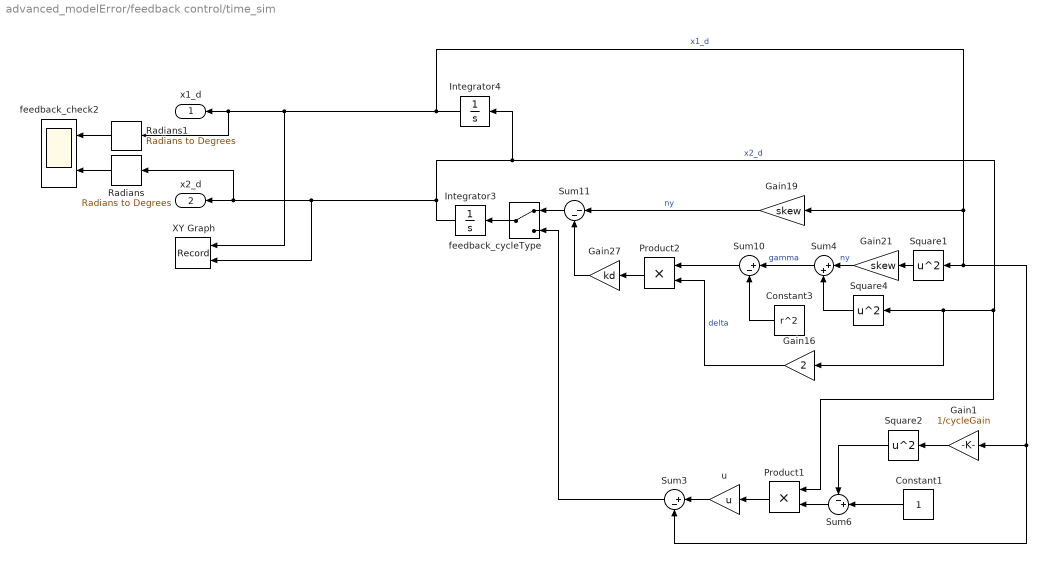
== system advanced_modelError/feedback control/time_sim ==
  Constant1 : Constant
  Constant3 : Constant  Value=r^2
  Gain1 : Gain  Gain=1/cycleGain
  Gain16 : Gain  Gain=2
  Gain19 : Gain  Gain=skew
  Gain21 : Gain  Gain=skew
  Gain27 : Gain  Gain=kd
  Integrator3 : Integrator  InitialCondition=0.00010472
  Integrator4 : Integrator  InitialCondition=0.00010472
  Product1 : Product
  Product2 : Product
  Radians : simulink_extras/Transformations/Radians to Degrees
  Radians1 : simulink_extras/Transformations/Radians to Degrees
  Square1 : Math  Operator=square
  Square2 : Math  Operator=square
  Square4 : Math  Operator=square
  Sum10 : Sum  Inputs=|+-
  Sum11 : Sum  Inputs=|--
  Sum3 : Sum  Inputs=|+-
  Sum4 : Sum  Inputs=|++
  Sum6 : Sum  Inputs=-+|
  XY Graph : Record  FileSettingsInternal="{\"entries\":[{\"content\":{\"excelSettings\":{\"content\":{},\"type\":\"Streamout.ExcelSettings\"}},\"type\":\"Streamout.FileSettingStorage\",\"uuid\":\"\"}],\"packageUris\":[\"http:\\/\\/schema.mathworks.com\\/mf0\\/streamout_blocks\\/R2020a\"],\"version\":\"1.0\"}"  Layout=[1 1]  SignalsInternal="{\"entries\":[{\"content\":{\"signals\":[{\"content\":{\"blockPath\":[],\"dimensions\":[1],\"domain\":\"\",\"lineColor\":\"#edb120\",\"port\":1,\"sid\":[\"\"],\"signalID\":31062,\"signalName\":\"x1_d\"},\"type\":\"RecordBlkView.Signal\",\"uuid\":\"\"},{\"content\":{\"blockPath\":[],\"dimensions\":[1],\"domain\":\"\",\"lineColor\":\"#7e2f8e\",\"port\":2,\"sid\":[\"\"],\"signalID\":31066,\"signalName\":\"x2_d\"},\"type\":\"RecordBlkView.Signal\",\"uuid\":\"\"}]},\"type\":\"RecordBlkView.InputSignals\",\"uuid\":\"\"}],\"packageUris\":[\"http:\\/\\/schema.mathworks.com\\/mf0\\/streamout_blocks\\/R2020a\"],\"version\":\"1.0\"}"  VisualizationBindings="{\"xyplotplugin\":{\"info\":[{\"series\":[],\"subplotID\":1}]}}"  CompatibilityTag=XY
  feedback_check2 : Scope  NumInputPorts=2
  feedback_cycleType : ManualSwitch
  u : Gain  Gain=u
  x1_d : Outport
  x2_d : Outport  Port=2
  wires:
  Square1/1 -> Gain21/1
  Square4/1 -> Sum4/2
  Integrator4/1 -> Sum3/2, Gain1/1, Square1/1, Gain19/1, XY Graph/1, Radians1/1, x1_d/1  "x1_d"
  Gain27/1 -> Sum11/2
  Gain16/1 -> Product2/2  "delta"
  Gain19/1 -> Sum11/1  "ny"
  Integrator3/1 -> Product1/1, Gain16/1, Square4/1, Integrator4/1, XY Graph/2, Radians/1, x2_d/1  "x2_d"
  Sum10/1 -> Product2/1
  Constant3/1 -> Sum10/2
  Gain21/1 -> Sum4/1  "ny"
  Sum4/1 -> Sum10/1  "gamma"
  Product2/1 -> Gain27/1
  Radians1/1 -> feedback_check2/1
  Radians/1 -> feedback_check2/2
  Square2/1 -> Sum6/1
  Gain1/1 -> Square2/1
  u/1 -> Sum3/1
  Product1/1 -> u/1
  Sum6/1 -> Product1/2
  Constant1/1 -> Sum6/2
  feedback_cycleType/1 -> Integrator3/1
  Sum11/1 -> feedback_cycleType/1
  Sum3/1 -> feedback_cycleType/2

== matlab function advanced_modelError/feedback control/MATLAB Function ==
  data: disable input; realValues input; outError output
function outError = approxLimitSimu(disable, realValues)
    outError = [0; 0];
    cyclePoint = [0; 0];
    %temp = load('paperCycle.mat');
    %cycleValues = temp.paperCycle;
    %for n = 1:2
    %    cycleN = cycleValues(:, n);
    %    realValueN = realValues(n);
    %    [closestValueError,idx]=min(abs(cycleN-realValueN));
    %    outError(n) = closestValueError;
    %end
    %disp(length(cycleValues))
    coder.extrinsic('approxLimit');
    coder.extrinsic('gainScheduling');
    if disable ~= 1
        cyclePoint = approxLimit(realValues);
        % K = [0, 0];
        % Km = zeros(2);
        % Kr = zeros(2);
        % K = gainScheduling(realValues);
        % Km = [K(1), 0; 0, K(2)];
        % outError = Km*(cyclePoint - realValues);
    end

== matlab function advanced_modelError/feedback control/Gain scheduling ==
  data: xv input; x input; e output
function e   = fcn(xv, x)
    K = [0, 0];
    Km = zeros(2);
    Kr = zeros(2);
    e = [0; 0];
    coder.extrinsic('gainScheduling');
    % K = gainScheduling(x);
    % Km = [K(1), 0; 0, K(2)];
    %Kr = 1;
    %K = 50*eye(2);
    %K = [5, 0; 0, 50];
    
    %e = Kr*xv - K*x;
    e = Km*(xv - x);
